simulink model "canonical_controlled_form"  (R2021b)
settings: Solver=VariableStepAuto  StartTime=0.0  StopTime=10.0  RelTol=1e-3
settings Model: Creator=den  LastModifiedBy=den

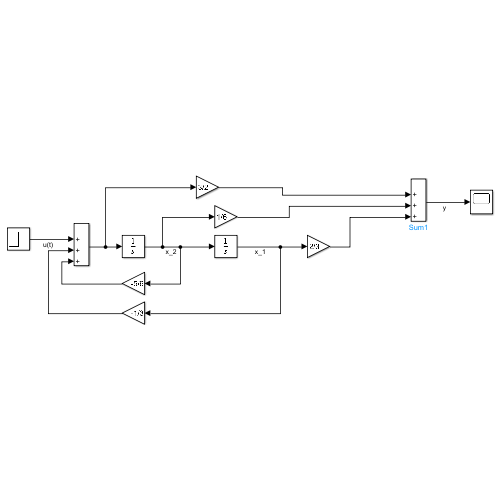
[thumbnail: Simulink's stored preview of the top-level diagram]
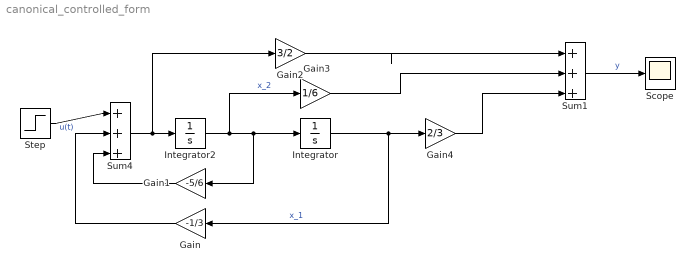
== system canonical_controlled_form ==
  Gain : Gain  Gain=-1/3
  Gain1 : Gain  Gain=-5/6
  Gain2 : Gain  Gain=3/2
  Gain3 : Gain  Gain=1/6
  Gain4 : Gain  Gain=2/3
  Integrator : Integrator
  Integrator2 : Integrator
  Scope : Scope
  Step : Step  Time=0  SampleTime=0
  Sum1 : Sum  Inputs=|+++
  Sum4 : Sum  Inputs=|+++
  wires:
  Step/1 -> Sum4/1  "u(t)"
  Gain/1 -> Sum4/2
  Sum4/1 -> Gain2/1, Integrator2/1
  Integrator2/1 -> Gain3/1, Integrator/1, Gain1/1  "x_2"
  Integrator/1 -> Gain4/1, Gain/1  "x_1"
  Gain1/1 -> Sum4/3
  Gain2/1 -> Sum1/1
  Gain3/1 -> Sum1/2
  Gain4/1 -> Sum1/3
  Sum1/1 -> Scope/1  "y"
